simulink model "GFo_29bus"  (R2019a)
settings: Solver=ode1  StartTime=0.0  StopTime=4.5  FixedStep=Time_Step  RelTol=1e-3  EnableMultiTasking=on
PreLoadFcn:
  | Init_29bus;
InitFcn:
  | Init_29bus;
undefined symbols (not defined in the file): D1, D11, Delta, Time_Step, VSC01_Delta_P_Time_Step, VSC01_Delta_P_Value
libraries: powerlib x169, sps_avr x6, GFo_Lib x1
(part 1 of 5)
Description:
  | Copyright 2008-2017 The MathWorks, Inc.
settings Model: Creator=MathWorks  LastModifiedBy=fcolas
settings DataIOCC: SaveFormat=StructureWithTime  SignalLoggingSaveFormat=ModelDataLogs  SaveOutput=off  SignalLogging=off  DSMLogging=off  SaveTime=off  ReturnWorkspaceOutputs=off
settings OptimizationCC: ExpressionDepthLimit=2147483647  LifeSpan=inf
settings DebuggingCC: UnderspecifiedInitializationDetection=Classic  MergeDetectMultiDrivingBlocksExec=none  SolverPrmCheckMsg=warning  FcnCallInpInsideContextMsg=warning  UnconnectedInputMsg=none  UnconnectedOutputMsg=none  UnconnectedLineMsg=none  StateNameClashWarn=warning  SFUnexpectedBacktrackingDiag=warning  SFNoUnconditionalDefaultTransitionDiag=warning  SFExecutionAtInitializationDiag=none  ArithmeticOperatorsInVariantConditions=warning
settings HardwareCC: ProdBitPerPointer=32  ProdBitPerSizeT=32  ProdBitPerPtrDiffT=32  ProdLargestAtomicFloat=None  ProdIntDivRoundTo=Undefined  ProdEndianess=Unspecified  ProdWordSize=32  ProdHWDeviceType=32-bit Generic
settings ModelReferenceCC: PropagateSignalLabelsOutOfModel=off
settings SFSimCC: SimUseLocalCustomCode=off
settings RTWCC: RTWUseLocalCustomCode=off
settings CodeAppCC: StateflowObjectComments=on
settings GRTTargetCC: TargetLangStandard=C89/C90 (ANSI)  CombineOutputUpdateFcns=off  GRTInterface=on
settings ConfigComp: CovMetricSettings=dw  CovSaveCumulativeToWorkspaceVar=on  CovSaveSingleToWorkspaceVar=on  CovExternalEMLEnable=off  CovSFcnEnable=off
settings SimscapeCC: SimscapeNormalizeSystem=off

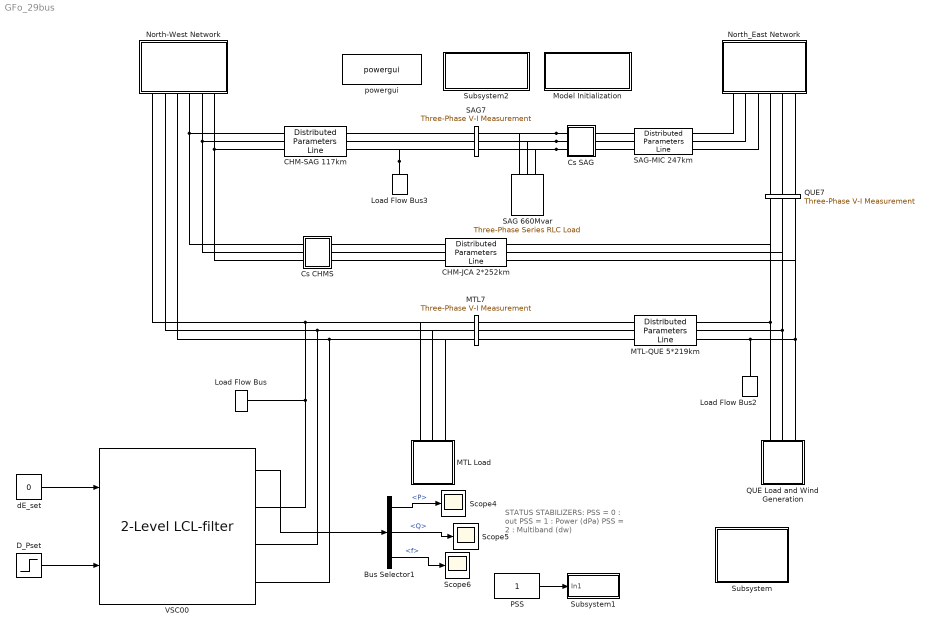
== system GFo_29bus ==
  note: STATUS STABILIZERS:
      | PSS = 0 :  out
      | PSS = 1 :  Power (dPa)
      | PSS = 2 :  Multiband (dw)
  Bus Selector1 : BusSelector  OutputSignals=P,Q,f
  CHM-JCA 2*252km : powerlib/Elements/Distributed Parameters Line  Phases=3  Length=252  Frequency=60  Resistance="[0.01273  0.3864]/2"  Inductance="[0.9337e-3  4.1264e-3]/2"  Capacitance=[12.74e-9 7.751e-9]*2  x1=[-0.00144 -3.19600605904016e-08 0 0;-0.0014 -3.19816909359179e-08 0 0;-0.00136 -3.19960489207136e-08 0 0;-0.00132 -3.2003131279907e-08 0 0;-0.00128 -3.20029364030306e-08 0 0;-0.00124 -3.19954643343978e-08 0 0;-0.0012 -3.19807167730924e-08 0 0;-0.00116 -3.19586970725827e-08 0 0;-0.00112 -3.19294102399589e-08 0 0;-0.00108 -3.18928629347939e-08 0 0;-0.00104 -3.184906346763e-08 0 0;-0.001 -3.17980217980881e-08 0 0;-0.00096 -3.17397495326038e-08 0 0;-0.00092 -3.16742599217877e-08 0 0;-0.00088 -3.16015678574126e-08 236947.551930455 -735006.025979769;-0.00084 -3.1521689869027e-08 248003.849356848 -731349.489711583;-0.0008 -3.14346441201967e-08 259003.752846592 -727526.650876326;-0.00076 -3.13404504043743e-08 269944.761116491 -723538.378754583;-0.00072 -3.12391301403984e-08 280824.386275617 -719385.58024504;-0.00068 -3.11307063676234e-08 291640.154391031 -715069.199658266;-0.00064 -3.10152037406802e-08 302389.606050334 -710590.218501984;-0.0006 -3.08926485238701e-08 313070.296920917 -705949.655257884;-0.00056 -3.07630685851926e-08 323679.798305784 -701148.565150029;-0.00052 -3.06264933900081e-08 334215.697695812 -696188.039904907;-0.00048 -3.04829539943384e-08 344675.599318338 -691069.207503179;-0.00044 -3.03324830378042e-08 355057.124681934 -685793.231923193;-0.0004 -3.01751147362034e-08 365357.913117259 -680361.312876297;-0.00036 -3.00108848737306e-08 375575.622313855 -674774.685534038;-0.00032 -2.98398307948405e-08 385707.928852762 -669034.620247298;-0.00028 -2.96619913957553e-08 395752.528734852 -663142.422257422;-0.00024 -2.94774071156208e-08 405707.137904732 -657099.431399422;-0.0002 -2.92861199273106e-08 415569.492770122 -650907.021797306;-0.00016 -2.90881733278817e-08 425337.350716574 -644566.601551616;-0.00012 -2.88836123286837e-08 435008.490617427 -638079.61241924;-8e-05 -2.86724834451239e-08 444580.713338866 -631447.529485563;-4e-05 -2.84548346860896e-08 454051.842239994 -624671.860829052]  x2=[-0.00144 -1.99708646271009e-08 0 0;-0.0014 -1.99485959351421e-08 0 0;-0.00136 -1.9921791104497e-08 0 0;-0.00132 -1.9890456230353e-08 0 0;-0.00128 -1.98545984379901e-08 0 0;-0.00124 -1.98142258811612e-08 0 0;-0.0012 -1.97693477402376e-08 0 0;-0.00116 -1.97199742201214e-08 0 0;-0.00112 -1.96661165479254e-08 0 0;-0.00108 -1.96077869704197e-08 0 0;-0.00104 -1.95449987512473e-08 0 0;-0.001 -1.94777661679078e-08 0 0;-0.00096 -1.94061045085108e-08 0 0;-0.00092 -1.93300300682997e-08 0 0;-0.00088 -1.92495601459461e-08 28167.8544791851 -750122.429836286;-0.00084 -1.91647130396165e-08 39475.8227942449 -749612.370451288;-0.0008 -1.90755080428111e-08 50774.8146476263 -748931.855677631;-0.00076 -1.8981965439977e-08 62062.2607460202 -748081.040258507;-0.00072 -1.88841065018953e-08 73335.5944215226 -747060.117662004;-0.00068 -1.87819534808447e-08 84592.2522152727 -745869.320037117;-0.00064 -1.86755296055411e-08 95829.6744603617 -744508.918160956;-0.0006 -1.85648590758562e-08 107045.305863878 -742979.221377177;-0.00056 -1.8449967057314e-08 118236.596087961 -741280.577525637;-0.00052 -1.83308796753687e-08 129401.000329722 -739413.372863299;-0.00048 -1.8207624009464e-08 140535.979899915 -737378.031976401;-0.00044 -1.80802280868754e-08 151639.002800209 -735175.017683909;-0.0004 -1.79487208763371e-08 162707.544298945 -732804.830932275;-0.00036 -1.78131322814546e-08 173739.087505238 -730268.010681527;-0.00032 -1.76734931339053e-08 184731.123941295 -727565.133782713;-0.00028 -1.75298351864271e-08 195681.15411282 -724696.814846731;-0.00024 -1.73821911055983e-08 206586.688077383 -721663.706104573;-0.0002 -1.72305944644097e-08 217445.246010605 -718466.497259008;-0.00016 -1.70750797346303e-08 228254.358770052 -715105.915327759;-0.00012 -1.69156822789684e-08 239011.568456696 -711582.724478174;-8e-05 -1.67524383430309e-08 249714.428973821 -707897.725853471;-4e-05 -1.65853850470811e-08 260360.506583243 -704051.757390559]  x3=[-0.00144 -7.69933611892035e-11 0 0;-0.0014 -7.64742706604721e-11 0 0;-0.00136 -7.59377905420784e-11 0 0;-0.00132 -7.53840428249751e-11 0 0;-0.00128 -7.48131534266176e-11 0 0;-0.00124 -7.42252521623322e-11 0 0;-0.0012 -7.36204727157963e-11 0 0;-0.00116 -7.29989526086407e-11 0 0;-0.00112 -7.23608331691782e-11 0 0;-0.00108 -7.17062595002662e-11 0 0;-0.00104 -7.10353804463122e-11 0 0;-0.001 -7.03483485594278e-11 0 0;-0.00096 -6.96453200647394e-11 0 0;-0.00092 -6.89264548248638e-11 0 0;-0.00088 -6.81919163035575e-11 329.831041715847 -923.135468477979;-0.00084 -6.74418715285459e-11 343.713540365703 -918.056958472584;-0.0008 -6.66764910535426e-11 357.517881520539 -912.769690231818;-0.00076 -6.58959489194672e-11 371.24092619222 -907.274866034884;-0.00072 -6.51004226148701e-11 384.87955387873 -901.573735357418;-0.00068 -6.42900930355724e-11 398.430663273748 -895.667594587374;-0.00064 -6.34651444435326e-11 411.891172971858 -889.557786730228;-0.0006 -6.26257644249465e-11 425.258022169232 -883.2457011036;-0.00056 -6.17721438475917e-11 438.528171359633 -876.732773021327;-0.00052 -6.09044768174262e-11 451.698603025574 -870.020483467091;-0.00048 -6.00229606344503e-11 464.766322324469 -863.110358757651;-0.00044 -5.91277957478421e-11 477.728357769642 -856.003970195776;-0.0004 -5.82191857103772e-11 490.581761906011 -848.702933712943;-0.00036 -5.72973371321427e-11 503.32361198032 -841.208909501886;-0.00032 -5.63624596335555e-11 515.951010605743 -833.523601639085;-0.00028 -5.54147657976968e-11 528.461086420726 -825.648757697273;-0.00024 -5.44544711219723e-11 540.850994741912 -817.586168348051;-0.0002 -5.348179396911e-11 553.117918210993 -809.337666954711;-0.00016 -5.24969555175064e-11 565.259067435359 -800.905129155335;-0.00012 -5.15001797109327e-11 577.271681622377 -792.290472436302;-8e-05 -5.04916932076113e-11 589.153029207173 -783.495655696258;-4e-05 -4.94717253286763e-11 600.900408473766 -774.522678800688]  x4=[-0.00144 -4.78587088598672e-11 0 0;-0.0014 -4.8966645663073e-11 0 0;-0.00136 -5.00634478733254e-11 0 0;-0.00132 -5.11488660872601e-11 0 0;-0.00128 -5.22226534901357e-11 0 0;-0.00124 -5.32845659119566e-11 0 0;-0.0012 -5.43343618829956e-11 0 0;-0.00116 -5.5371802688702e-11 0 0;-0.00112 -5.63966524239831e-11 0 0;-0.00108 -5.7408678046847e-11 0 0;-0.00104 -5.84076494313944e-11 0 0;-0.001 -5.93933394201472e-11 0 0;-0.00096 -6.03655238757023e-11 0 0;-0.00092 -6.13239817316981e-11 0 0;-0.00088 -6.22684950430836e-11 -191.737879033599 -10272.54825288;-0.00084 -6.31988490356769e-11 -36.8152546194894 -10274.2711335707;-0.0008 -6.41148321550032e-11 118.115741266039 -10273.6577336072;-0.00076 -6.50162361144002e-11 273.019878650591 -10270.7081924713;-0.00072 -6.59028559423809e-11 427.861933669161 -10265.4231808633;-0.00068 -6.67744900292424e-11 582.606696573739 -10257.8039005491;-0.00064 -6.76309401729099e-11 737.218979739702 -10247.8520840876;-0.0006 -6.84720116240064e-11 891.663625667178 -10235.5699944358;-0.00056 -6.92975131301371e-11 1045.90551497556 -10220.960424435;-0.00052 -7.01072569793784e-11 1199.90957438934 -10204.0266961756;-0.00048 -7.09010590429617e-11 1353.64078471348 -10184.7726602412;-0.00044 -7.16787388171434e-11 1507.06418879648 -10163.2026948337;-0.0004 -7.24401194642492e-11 1660.14489947931 -10139.321704777;-0.00036 -7.31850278528858e-11 1812.84810752848 -10113.1351204025;-0.00032 -7.39132945973095e-11 1965.13908955134 -10084.6488963136;-0.00028 -7.46247540959428e-11 2116.98321589187 -10053.8695100319;-0.00024 -7.53192445690312e-11 2268.3459585052 -10020.8039605246;-0.0002 -7.59966080954301e-11 2419.19289880894 -9985.45976661232;-0.00016 -7.66566906485149e-11 2569.48973550972 -9947.84496526009;-0.00012 -7.72993421312054e-11 2719.20229240298 -9907.96810974931;-8e-05 -7.79244164100964e-11 2868.29652614436 -9865.83826773306;-4e-05 -7.85317713486873e-11 3016.73853399082 -9821.46501917409]  x5=0.00142516474882927  V1=ones(3,3)  V2=ones(3,3)  I1=ones(3,3)  I2=ones(3,3)  nHarmo=1  Measurements=None  Decoupling=off  VsMag0=0  VrMag0=0  VsAngle0=0  VrAngle0=0  IsMag0=0  IrMag0=0  IsAngle0=0  IrAngle0=0
      settings: AttributesFormatString=\n
  CHM-SAG 117km : powerlib/Elements/Distributed Parameters Line  Phases=3  Length=117  Frequency=60  Resistance="[0.01273  0.3864]"  Inductance="[0.9337e-3  4.1264e-3]"  Capacitance=[12.74e-9 7.751e-9]  x1=[-0.00068 -3.03380786364724e-08 0 0;-0.00064 -3.02440322105761e-08 0 0;-0.0006 -3.01431085525686e-08 0 0;-0.00056 -3.00353306116193e-08 0 0;-0.00052 -2.99207228955026e-08 0 0;-0.00048 -2.97993114650248e-08 0 0;-0.00044 -2.96711239280981e-08 285915.250875642 -721016.735543736;-0.0004 -2.95361894334631e-08 296755.036613392 -716623.402960289;-0.00036 -2.93945386640601e-08 307527.342814922 -712067.116394906;-0.00032 -2.92462038300527e-08 318229.719950699 -707348.911907859;-0.00028 -2.90912186615028e-08 328859.734392455 -702469.862378162;-0.00024 -2.89296184007012e-08 339414.968966577 -697431.077259603;-0.0002 -2.87614397941538e-08 349893.023503745 -692233.702328464;-0.00016 -2.85867210842252e-08 360291.515384717 -686878.919422984;-0.00012 -2.84055020004435e-08 370608.080082112 -681367.94617462;-8e-05 -2.82178237504655e-08 380840.371698085 -675702.035731162;-4e-05 -2.80237290107068e-08 390986.063497761 -669882.476471785]  x2=[-0.00068 -2.03559263742575e-08 0 0;-0.00064 -2.02730116097309e-08 0 0;-0.0006 -2.01854869371913e-08 0 0;-0.00056 -2.00933722589944e-08 0 0;-0.00052 -1.99966885212236e-08 0 0;-0.00048 -1.98954577089273e-08 0 0;-0.00044 -1.9789702841119e-08 332776.301409875 -689011.544371815;-0.0004 -1.96794479655438e-08 343128.151600731 -683915.224593623;-0.00036 -1.95647181532096e-08 353401.977408923 -678663.388391192;-0.00032 -1.94455394926862e-08 363595.442655062 -673257.229986786;-0.00028 -1.93219390841734e-08 373706.229433054 -667697.978694203;-0.00024 -1.91939450333382e-08 383732.038637179 -661986.898639247;-0.0002 -1.9061586444924e-08 393670.590484882 -656125.288472272;-0.00016 -1.89248934161323e-08 403519.625035179 -650114.481072883;-0.00012 -1.8783897029779e-08 413276.902702548 -643955.843246846;-8e-05 -1.86386293472267e-08 422940.204766191 -637650.775415293;-4e-05 -1.84891234010935e-08 432507.333874551 -631200.711296277]  x3=[-0.00068 -2.53056281828965e-11 0 0;-0.00064 -2.45024672055226e-11 0 0;-0.0006 -2.36937345784065e-11 0 0;-0.00056 -2.28796142003733e-11 0 0;-0.00052 -2.20602911953763e-11 0 0;-0.00048 -2.12359518704014e-11 0 0;-0.00044 -2.04067836731021e-11 1667.28750300292 -3842.30394709011;-0.0004 -1.95729751491762e-11 1725.03630670092 -3816.72583715085;-0.00036 -1.87347158994916e-11 1782.39285201884 -3790.27983667027;-0.00032 -1.78921965369727e-11 1839.34409657292 -3762.97195924081;-0.00028 -1.7045608643257e-11 1895.87709014127 -3734.80841443831;-0.00024 -1.61951447251309e-11 1951.97897760867 -3705.79560640998;-0.0002 -1.53409981707553e-11 2007.6370018897 -3675.94013241817;-0.00016 -1.44833632056908e-11 2062.83850682964 -3645.24878134021;-0.00012 -1.36224348487326e-11 2117.57094008228 -3613.72853212466;-8e-05 -1.27584088675646e-11 2171.8218559643 -3581.38655220437;-4e-05 -1.1891481734244e-11 2225.57891828527 -3548.23019586668]  x4=[-0.00068 -4.55030209021528e-11 0 0;-0.00064 -4.62034510762418e-11 0 0;-0.0006 -4.68933749839977e-11 0 0;-0.00056 -4.75726357426735e-11 0 0;-0.00052 -4.82410788942303e-11 0 0;-0.00048 -4.88985524404599e-11 0 0;-0.00044 -4.95449068775477e-11 212.800113436249 -1518.35731015853;-0.0004 -5.01799952300687e-11 235.671559779652 -1514.9757824875;-0.00036 -5.08036730844081e-11 258.489416442706 -1511.24976238813;-0.00032 -5.14157986216004e-11 281.248494841579 -1507.18009712526;-0.00028 -5.20162326495771e-11 303.943619758109 -1502.76771210566;-0.00024 -5.26048386348182e-11 326.569630516604 -1498.01361066765;-0.0002 -5.31814827333985e-11 349.121382157336 -1492.9188738529;-0.00016 -5.37460338214228e-11 371.59374660646 -1487.48466016061;-0.00012 -5.42983635248422e-11 393.981613842093 -1481.71220528413;-8e-05 -5.48383462486452e-11 416.279893056292 -1475.6028218299;-4e-05 -5.5365859205417e-11 438.483513812655 -1469.15789901905]  x5=0.000661683633385019  V1=ones(3,3)  V2=ones(3,3)  I1=ones(3,3)  I2=ones(3,3)  nHarmo=1  Measurements=None  Decoupling=off  VsMag0=0  VrMag0=0  VsAngle0=0  VrAngle0=0  IsMag0=0  IrMag0=0  IsAngle0=0  IrAngle0=0
      settings: AttributesFormatString=\n
  Cs CHMS : Subsystem  mask{Xc=33/2}
      mask prompts: Xc "Condensator Reactance at  60Hz  (ohm):"
      mask help: Series Compensation
      mask init:
      | Cs=1/Xc/(2*pi*60);
      mask Display: disp('Cs')
  Cs SAG : Subsystem  mask{Xc=22}
      mask prompts: Xc "Condensator Reactance at  60Hz  (ohm):"
      mask help: Series Compensation
      mask init:
      | Cs=1/Xc/(2*pi*60);
      mask Display: disp('Cs')
  D_Pset : Step  Time=VSC01_Delta_P_Time_Step  After=VSC01_Delta_P_Value  SampleTime=0
  Load Flow Bus : powerlib/Measurements/Load Flow Bus  LConnTagsString=a  Phases=single  Connectors=on one side  ID=BUS_1  Vbase=VSC01_Un2  Vref=1  Vangle=0  VLF=1  VLFb=1  VLFc=1  angleLF=-17.01  angleLFb=0  angleLFc=0
  Load Flow Bus2 : powerlib/Measurements/Load Flow Bus  LConnTagsString=a  Phases=single  Connectors=on one side  ID=QUE7  Vbase=735e3  Vref=1  Vangle=0  VLF=1.021  VLFb=1  VLFc=1  angleLF=-8.842  angleLFb=0  angleLFc=0
      settings: AttributesFormatString=%<ID>\n%<Vbase>V\n%<VLF>pu\n%<angleLF>deg.
  Load Flow Bus3 : powerlib/Measurements/Load Flow Bus  LConnTagsString=a  Phases=single  Connectors=on one side  ID=SAG7  Vbase=735e3  Vref=1  Vangle=0  VLF=1.041  VLFb=1  VLFc=1  angleLF=5.283  angleLFb=0  angleLFc=0
      settings: AttributesFormatString=%<ID>\n%<Vbase>V\n%<VLF>pu\n%<angleLF>deg.
  MTL Load : Subsystem
  MTL-QUE 5*219km : powerlib/Elements/Distributed Parameters Line  Phases=3  Length=219  Frequency=60  Resistance="[0.01273  0.3864]/5"  Inductance="[0.9337e-3  4.1264e-3]/5"  Capacitance=[12.74e-9 7.751e-9]*5  x1=[-0.00124 -1.25867854068197e-07 -175262.845803513 -713799.758659387;-0.0012 -1.25881992959478e-07 -164479.469159206 -716361.379291285;-0.00116 -1.25867507371121e-07 -153658.691302023 -718760.10552317;-0.00112 -1.25824400597023e-07 -142802.972783534 -720995.391905382;-0.00108 -1.25752682439292e-07 -131914.782100514 -723066.730153074;-0.00104 -1.2565236920602e-07 -120996.59513363 -724973.649261791;-0.001 -1.2552348370757e-07 -110050.894584442 -726715.715614573;-0.00096 -1.25366055251394e-07 -99080.1694108641 -728292.533080553;-0.00092 -1.25180119635364e-07 -88086.9142611932 -729703.743105038;-0.00088 -1.24965719139636e-07 -77073.6289068485 -730949.024791039;-0.00084 -1.24722902517035e-07 -66042.8176739451 -732028.094972237;-0.0008 -1.24451724981965e-07 -54996.9888738316 -732940.70827738;-0.00076 -1.24152248197861e-07 -43938.6542327221 -733686.657186073;-0.00072 -1.2382454026316e-07 -32870.3283205508 -734265.772075965;-0.00068 -1.2346867569582e-07 -21794.5279791811 -734677.921261326;-0.00064 -1.23084735416376e-07 -10713.7717500969 -734923.011022985;-0.0006 -1.22672806729535e-07 369.420698291617 -735000.985629643;-0.00056 -1.2223298330433e-07 11452.5291435991 -734911.827350547;-0.00052 -1.21765365152813e-07 22533.0333825417 -734655.556459522;-0.00048 -1.21270058607321e-07 33608.4138040097 -734232.231230357;-0.00044 -1.20747176296289e-07 44676.1519620054 -733641.94792356;-0.0004 -1.20196837118647e-07 55733.7311483156 -732884.840764464;-0.00036 -1.19619166216778e-07 66778.6369647899 -731961.081912707;-0.00032 -1.19014294948063e-07 77808.3578950928 -730870.881423087;-0.00028 -1.18382360855012e-07 88820.3858758011 -729614.487197794;-0.00024 -1.17723507633989e-07 99812.2168667156 -728192.184930039;-0.0002 -1.17037885102534e-07 110781.351420259 -726604.298039093;-0.00016 -1.16325649165298e-07 121725.295249826 -724851.187596741;-0.00012 -1.15586961778592e-07 132641.559796968 -722933.25224518;-8e-05 -1.14821990913557e-07 143527.662797265 -720850.92810637;-4e-05 -1.14030910517971e-07 154381.128844771 -718604.688682862]  x2=[-0.00124 -1.98142258811612e-08 -73583.3206392189 -747036.13816367;-0.0012 -1.97693477402376e-08 -62310.3261187054 -748060.740678712;-0.00116 -1.97199742201214e-08 -51023.1627673739 -748915.240632326;-0.00112 -1.96661165479254e-08 -39724.3971888341 -749599.443718591;-0.00108 -1.96077869704197e-08 -28416.5986249423 -750113.194355623;-0.00104 -1.95449987512473e-08 -17102.3383715773 -750456.37572096;-0.001 -1.94777661679078e-08 -5784.18919395105 -750628.909778118;-0.00096 -1.94061045085108e-08 5535.27525841725 -750630.757294341;-0.00092 -1.93300300682997e-08 16853.481036926 -750461.917849519;-0.00088 -1.92495601459461e-08 28167.8544791852 -750122.429836286;-0.00084 -1.91647130396165e-08 39475.8227942449 -749612.370451288;-0.0008 -1.90755080428111e-08 50774.8146476264 -748931.855677631;-0.00076 -1.8981965439977e-08 62062.2607460202 -748081.040258507;-0.00072 -1.88841065018953e-08 73335.5944215226 -747060.117662004;-0.00068 -1.87819534808447e-08 84592.2522152728 -745869.320037117;-0.00064 -1.86755296055411e-08 95829.6744603617 -744508.918160956;-0.0006 -1.85648590758562e-08 107045.305863878 -742979.221377177;-0.00056 -1.8449967057314e-08 118236.596087961 -741280.577525637;-0.00052 -1.83308796753687e-08 129401.000329722 -739413.372863299;-0.00048 -1.8207624009464e-08 140535.979899915 -737378.031976401;-0.00044 -1.80802280868754e-08 151639.002800209 -735175.017683909;-0.0004 -1.79487208763371e-08 162707.544298945 -732804.830932275;-0.00036 -1.78131322814546e-08 173739.087505238 -730268.010681527;-0.00032 -1.76734931339053e-08 184731.123941295 -727565.133782713;-0.00028 -1.75298351864271e-08 195681.15411282 -724696.814846731;-0.00024 -1.73821911055983e-08 206586.688077383 -721663.706104573;-0.0002 -1.72305944644097e-08 217445.246010605 -718466.497259008;-0.00016 -1.70750797346303e-08 228254.358770052 -715105.915327759;-0.00012 -1.69156822789684e-08 239011.568456696 -711582.724478174;-8e-05 -1.67524383430309e-08 249714.428973821 -707897.725853471;-4e-05 -1.65853850470811e-08 260360.506583243 -704051.757390559]  x3=[-0.00124 -5.10144217917009e-10 -7027.03988727101 -19339.1228874643;-0.0012 -4.91343394355244e-10 -6734.62515238683 -19442.8845645399;-0.00116 -4.72430843542768e-10 -6440.67902181993 -19542.2250973339;-0.00112 -4.53410866030541e-10 -6145.26833638552 -19637.1218966656;-0.00108 -4.34287786797427e-10 -5848.46026992595 -19727.5533838215;-0.00104 -4.15065954266734e-10 -5550.32231403597 -19813.4989954609;-0.001 -3.95749739317417e-10 -5250.92226271573 -19894.9391882932;-0.00096 -3.76343534290179e-10 -4950.32819695497 -19971.8554435207;-0.00092 -3.56851751988693e-10 -4648.60846925203 -20044.2302710503;-0.00088 -3.37278824676162e-10 -4345.83168807107 -20112.0472134703;-0.00084 -3.17629203067469e-10 -4042.06670224111 -20175.2908497929;-0.0008 -2.97907355317116e-10 -3737.38258530035 -20233.9467989606;-0.00076 -2.78117766003207e-10 -3431.84861978952 -20288.0017231163;-0.00072 -2.58264935107695e-10 -3125.53428149754 -20337.4433306364;-0.00068 -2.38353376993122e-10 -2818.50922366341 -20382.2603789258;-0.00064 -2.18387619376091e-10 -2510.84326113761 -20422.4426769741;-0.0006 -1.9837220229771e-10 -2202.60635450682 -20457.9810876734;-0.00056 -1.78311677091215e-10 -1893.86859418547 -20488.8675298954;-0.00052 -1.58210605347044e-10 -1584.70018447784 -20515.0949803296;-0.00048 -1.38073557875567e-10 -1275.17142761413 -20536.6574750799;-0.00044 -1.17905113667725e-10 -965.352707764394 -20553.550111021;-0.0004 -9.77098588538048e-11 -655.314475033757 -20565.7690469131;-0.00036 -7.74923856605955e-11 -345.127229442688 -20573.3115042756;-0.00032 -5.72572913671529e-11 -34.8615048958939 -20576.1757680186;-0.00028 -3.70091772594193e-11 275.41214685648 -20574.3611868334;-0.00024 -1.67526475839304e-11 585.623172261712 -20567.8681733401;-0.0002 3.50769149915035e-12 895.701032007771 -20556.6982039939;-0.00016 2.37672329634333e-11 1205.57521706335 -20540.8538187495;-0.00012 4.40213699639002e-11 1515.175264711 -20520.3386204835;-8e-05 6.42654968844614e-11 1824.43077456978 -20495.1572741751;-4e-05 8.44950103852332e-11 2133.27142460364 -20465.3155058452]  x4=[-0.00124 -4.08867860944578e-10 -1381.07232417721 -6777.19407549483;-0.0012 -4.30955175950684e-10 -1278.7208894892 -6797.24853422087;-0.00116 -4.52944495466178e-10 -1176.07868469815 -6815.7573572472;-0.00112 -4.74830819309429e-10 -1073.16904975626 -6832.71633582708;-0.00108 -4.96609170719137e-10 -970.015385427081 -6848.12161363503;-0.00104 -5.18274597485997e-10 -866.641147964308 -6861.96968764373;-0.001 -5.398221730788e-10 -763.069843778083 -6874.25740892056;-0.00096 -5.61246997764672e-10 -659.325024089817 -6884.98198334367;-0.00092 -5.82544199723241e-10 -555.43027957685 -6894.14097223733;-0.00088 -6.03708936154439e-10 -451.409235008133 -6901.73229292644;-0.00084 -6.24736394379721e-10 -347.285543872164 -6907.75421921014;-0.0008 -6.45621792936417e-10 -243.08288299838 -6912.20538175433;-0.00076 -6.66360382665005e-10 -138.824947173261 -6915.08476840304;-0.00072 -6.86947447789023e-10 -34.5354437523297 -6916.39172440855;-0.00068 -7.07378306987395e-10 69.76191273069 -6916.12595258036;-0.00064 -7.27648314458929e-10 174.043405956356 -6914.28751335268;-0.0006 -7.47752860978728e-10 278.285323212394 -6910.87682477074;-0.00056 -7.67687374946285e-10 382.463960785763 -6905.89466239571;-0.00052 -7.87447323425034e-10 486.555629352679 -6899.34215912835;-0.00048 -8.07028213173093e-10 590.536659365357 -6891.2208049514;-0.00044 -8.2642559166499e-10 694.383406434267 -6881.53244659076;-0.0004 -8.45635048104134e-10 798.072256704661 -6870.27928709557;-0.00036 -8.64652214425785e-10 901.579632226162 -6857.46388533727;-0.00032 -8.8347276629032e-10 1004.88199631419 -6843.08915542768;-0.00028 -9.02092424066543e-10 1107.95585890198 -6827.15836605644;-0.00024 -9.20506953804849e-10 1210.77778188207 -6809.67513974767;-0.0002 -9.38712168199972e-10 1313.32438443586 -6790.64345203625;-0.00016 -9.56703927543156e-10 1415.57234835025 -6770.06763056386;-0.00012 -9.7447814066348e-10 1517.49842332001 -6747.95235409485;-8e-05 -9.92030765858159e-10 1619.07943223465 -6724.30265145239;-4e-05 -1.00935781181159e-09 1720.29227644875 -6699.1239003749]  x5=0.00123853603172068  V1=ones(3,3)  V2=ones(3,3)  I1=ones(3,3)  I2=ones(3,3)  nHarmo=1  Measurements=None  Decoupling=off  VsMag0=0  VrMag0=0  VsAngle0=0  VrAngle0=0  IsMag0=0  IrMag0=0  IsAngle0=0  IrAngle0=0
      settings: AttributesFormatString=\n
  MTL7 : powerlib/Measurements/Three-Phase V-I Measurement  VoltageMeasurement=phase-to-ground  SetLabelV=on  LabelV=Vabc_MTL7  Vpu=on  VpuLL=off  CurrentMeasurement=no  SetLabelI=off  LabelI=A1  Ipu=off  Pbase=100e6  Vbase=735e3  OutputType=Magnitude  PhasorSimulation=off  PSBequivalent=0
  Model Initialization : Subsystem  mask(Model Functions){InitFcnX=Init_29bus;, prel=on, posl=off, inif=on, strf=off}
      mask prompts: InitFcnX "Initialisation"; prel "Preload Function"; posl "PostLoad Function"; inif "InitFcn"; strf "StartFcn"
      mask init:
      | currentBlock = gcb;
      | root = bdroot(currentBlock);
      | 
      | if ~strcmp(get_param(root,'BlockDiagramType'),'library')
      |     if prel==1
      |         set_param(root, 'PreLoadFcn', InitFcnX);
      |     else
      |         set_param(root, 'PreLoadFcn', '');
      |     end
      |     if inif==1
      |         set_param(root, 'InitFcn', InitFcnX);
      |     else
      |         set_param(root, 'InitFcn', '');
      |     end
      |     if strf==1
      |         set_param(root, 'StartFcn', InitFcnX);
      |     else
      |         set_param(root, 'StartFcn', '');
      |     end
      |     if posl==1
      |         set_param(root, 'PostLoadFcn', InitFcnX);
      |     else
      |         set_param(root, 'PostLoadFcn', '');
      |     end
      | end
      | 
      | pos = get_param(currentBlock, 'Position');
      | width = pos(3) - pos(1); height = pos(4) - pos(2);
      | txt = [ upper(root) '\n' '- InitFcn. . . . . '  get_param(root, 'InitFcn') ];
      settings: CopyFcn=set_param(gcb,'LinkStatus','none')
      mask Display:
      | %text(5, height*0.5, txt, 'horizontalAlignment', 'left', 'verticalAlignment', 'middle') ;
      | color('blue'),disp('Initialization Function\nParameters')
  North-West Network : Subsystem
  North_East Network : Subsystem
  PSS : Constant
  QUE Load and Wind Generation : Subsystem
  QUE7 : powerlib/Measurements/Three-Phase V-I Measurement  VoltageMeasurement=no  SetLabelV=on  LabelV=Vabc_QUE7  Vpu=on  VpuLL=off  CurrentMeasurement=no  SetLabelI=off  LabelI=A1  Ipu=off  Pbase=100e6  Vbase=735e3  OutputType=Magnitude  PhasorSimulation=off  PSBequivalent=0
  SAG 660Mvar : powerlib/Elements/Three-Phase Series RLC Load  LConnTagsString=A|B|C  Configuration=Y (grounded)  NominalVoltage=735e3  Vabc=[1e3 1e3 1e3]  Vabcp=[1e3 1e3 1e3]  NominalFrequency=60  UnbalancedPower=off  ActivePower=2200000  InductivePower=660e6  CapacitivePower=0  Pabc=[10e3 9e3 11e3]  QLabc=[100 90 110]  QCabc=[100 90 110]  Pabcp=[10e3 9e3 11e3]  QLabcp=[100 90 110]  QCabcp=[100 90 110]  Measurements=None  LoadType=constant Z
  SAG-MIC 247km : powerlib/Elements/Distributed Parameters Line  Phases=3  Length=247  Frequency=60  Resistance="[0.01273  0.3864]/1"  Inductance="[0.9337e-3  4.1264e-3]/1"  Capacitance=[12.74e-9 7.751e-9]*1  x1=[-0.0014 -2.0715212238375e-08 36522.5847829561 -754650.708753614;-0.00136 -2.07364597068543e-08 47897.8850362566 -754014.151844709;-0.00132 -2.07529918832199e-08 59262.2937235537 -753206.138620016;-0.00128 -2.07648050081973e-08 70613.2266763144 -752226.852814774;-0.00124 -2.0771896395584e-08 81948.1027902712 -751076.51711013;-0.0012 -2.07742644328595e-08 93264.3446123441 -749755.393082503;-0.00116 -2.07719085815526e-08 104559.378926729 -748263.781144104;-0.00112 -2.07648293773636e-08 115830.637340029 -746602.020474625;-0.00108 -2.07530284300425e-08 127075.556865277 -744770.488944111;-0.00104 -2.07365084230228e-08 138291.580504748 -742769.603027039;-0.001 -2.07152731128118e-08 149476.157831388 -740599.817707611;-0.00096 -2.06893273281358e-08 160626.745568764 -738261.626376297;-0.00092 -2.06586769688425e-08 171740.808169384 -735755.560717642;-0.00088 -2.06233290045594e-08 182815.818391256 -733082.190589366;-0.00084 -2.05832914731087e-08 193849.257872562 -730242.123892781;-0.0008 -2.05385734786797e-08 204838.617704313 -727236.006434563;-0.00076 -2.04891851897588e-08 215781.399000851 -724064.521779898;-0.00072 -2.0435137836817e-08 226675.113468075 -720728.391097046;-0.00068 -2.03764437097562e-08 237517.28396926 -717228.372993356;-0.00064 -2.03131161551147e-08 248305.445088332 -713565.263342761;-0.0006 -2.02451695730325e-08 259037.143690486 -709739.895104807;-0.00056 -2.01726194139762e-08 269709.939480006 -705753.138135243;-0.00052 -2.00954821752264e-08 280321.405555168 -701605.898988222;-0.00048 -2.00137753971261e-08 290869.128960095 -697299.120710163;-0.00044 -1.99275176590919e-08 301350.711233445 -692833.782625306;-0.0004 -1.98367285753896e-08 311763.768953799 -688210.900113024;-0.00036 -1.9741428790674e-08 322105.934281629 -683431.524376934;-0.00032 -1.96416399752941e-08 332374.855497726 -678496.742205864;-0.00028 -1.95373848203662e-08 342568.197537962 -673407.675726722;-0.00024 -1.94286870326134e-08 352683.64252426 -668165.482149341;-0.0002 -1.93155713289752e-08 362718.890291662 -662771.353503333;-0.00016 -1.91980634309872e-08 372671.658911367 -657226.516367035;-0.00012 -1.9076190058932e-08 382539.685209618 -651532.231588595;-8e-05 -1.89499789257635e-08 392320.725282335 -645689.793999266;-4e-05 -1.88194587308049e-08 402012.555005352 -639700.532118974]  x2=[-0.0014 -8.27139318429975e-09 154421.725077414 -749560.143874635;-0.00136 -8.30049042152564e-09 165706.858590059 -747146.344688553;-0.00132 -8.32770019881005e-09 176954.311792055 -744562.650866804;-0.00128 -8.35301632888428e-09 188161.527109539 -741809.649919084;-0.00124 -8.37643305507867e-09 199325.956118394 -738887.967854065;-0.0012 -8.39794505263161e-09 210445.060123741 -735798.269037055;-0.00116 -8.41754742990038e-09 221516.310737217 -732541.25603892;-0.00112 -8.43523572947343e-09 232537.190451907 -729117.669476329;-0.00108 -8.45100592918398e-09 243505.193214803 -725528.287843341;-0.00104 -8.46485444302459e-09 254417.824996662 -721773.927334388;-0.001 -8.47677812196266e-09 265272.604359122 -717855.441658672;-0.00096 -8.48677425465641e-09 276067.063018965 -713773.721846044;-0.00092 -8.49484056807148e-09 286798.746409378 -709529.696044391;-0.00088 -8.50097522799776e-09 297465.214238104 -705124.329308581;-0.00084 -8.50517683946648e-09 308064.041042344 -700558.62338102;-0.0008 -8.50744444706742e-09 318592.816740282 -695833.616463862;-0.00076 -8.50777753516618e-09 329049.14717912 -690950.382982933;-0.00072 -8.50617602802139e-09 339430.654679489 -685910.033343417;-0.00068 -8.50264028980196e-09 349734.978576109 -680713.713677354;-0.00064 -8.49717112450428e-09 359959.775754587 -675362.605583027;-0.0006 -8.48976977576937e-09 370102.721184219 -669857.925856268;-0.00056 -8.48043792660011e-09 380161.508446684 -664200.926213779;-0.00052 -8.46917769897852e-09 390133.850260501 -658392.893008494;-0.00048 -8.45599165338326e-09 400017.47900114 -652435.146937077;-0.00044 -8.44088278820739e-09 409810.147216658 -646329.042739607;-0.0004 -8.42385453907655e-09 419509.628138751 -640075.968891523;-0.00036 -8.40491077806776e-09 429113.716189102 -633677.347287893;-0.00032 -8.38405581282889e-09 438620.227480911 -627134.632920091;-0.00028 -8.3612943855992e-09 448027.000315491 -620449.313544941;-0.00024 -8.33663167213097e-09 457331.895673819 -613622.909346418;-0.0002 -8.31007328051254e-09 466532.797702933 -606656.972589968;-0.00016 -8.28162524989314e-09 475627.614197057 -599553.087269538;-0.00012 -8.25129404910961e-09 484614.277073351 -592312.868747389;-8e-05 -8.21908657521544e-09 493490.742842173 -584937.963386775;-4e-05 -8.18501015191245e-09 502254.993071756 -577430.048177577]  x3=[-0.0014 -1.78924563946058e-11 -207.547752866833 -4152.7477084931;-0.00136 -1.75997703945032e-11 -144.904646865292 -4155.40507498295;-0.00132 -1.73030823583868e-11 -82.2285907966585 -4157.11753819343;-0.00128 -1.70024597505576e-11 -19.5338366555868 -4157.88470872519;-0.00124 -1.66979709300041e-11 43.1653593114872 -4157.70641213025;-0.0012 -1.63896851348582e-11 105.854739848097 -4156.58268895172;-0.00116 -1.60776724666513e-11 168.520049929717 -4154.51379471457;-0.00112 -1.57620038743735e-11 231.147040005238 -4151.50019986751;-0.00108 -1.54427511383403e-11 293.721469237189 -4147.542589676;-0.00104 -1.51199868538709e-11 356.229108739981 -4142.64186406649;-0.001 -1.47937844147802e-11 418.655744815435 -4136.79913742171;-0.00096 -1.44642179966896e-11 480.987182184852 -4130.01573832732;-0.00092 -1.41313625401608e-11 543.209247216896 -4122.29320926977;-0.00088 -1.3795293733654e-11 605.307791150561 -4113.63330628557;-0.00084 -1.34560879963177e-11 667.268693312469 -4104.03799856199;-0.0008 -1.31138224606114e-11 729.077864327799 -4093.50946798926;-0.00076 -1.27685749547663e-11 790.72124932408 -4082.05010866442;-0.00072 -1.2420423985088e-11 852.184831127155 -4069.66252634697;-0.00068 -1.20694487181047e-11 913.45463344856 -4056.34953786631;-0.00064 -1.17157289625654e-11 974.516724063616 -4042.11417048121;-0.0006 -1.13593451512922e-11 1035.3572179795 -4026.95966119144;-0.00056 -1.10003783228903e-11 1095.96228059255 -4010.88945600175;-0.00052 -1.06389101033211e-11 1156.31813083417 -3993.90720913819;-0.00048 -1.02750226873404e-11 1216.4110443045 -3976.01678221727;-0.00044 -9.90879881980864e-12 1276.22735639323 -3957.22224336777;-0.0004 -9.54032177687509e-12 1335.75346538684 -3937.52786630577;-0.00036 -9.16967534704172e-12 1394.97583556147 -3916.93812936277;-0.00032 -8.79694381211034e-12 1453.88100026085 -3895.45771446738;-0.00028 -8.4222119280177e-12 1512.45556495851 -3873.09150608072;-0.00024 -8.04556490556269e-12 1570.68621030356 -3849.84459008569;-0.0002 -7.66708839103015e-12 1628.55969514941 -3825.72225263053;-0.00016 -7.28686844671565e-12 1686.06285956467 -3800.72997892674;-0.00012 -6.90499153135564e-12 1743.18262782567 -3774.87345200184;-8e-05 -6.52154448046751e-12 1799.90601138966 -3748.15855140708;-4e-05 -6.13661448660393e-12 1856.22011184838 -3720.59135188047]  x4=[-0.0014 -1.89201204911383e-11 11.9349515108093 -1468.59968146629;-0.00136 -1.94615873981848e-11 34.0788908853198 -1468.2525709345;-0.00132 -1.99986289080864e-11 56.215081013927 -1467.57159242976;-0.00128 -2.05311229022353e-11 78.3384883178897 -1466.55690080069;-0.00124 -2.1058948296089e-11 100.444082125171 -1465.20872677942;-0.0012 -2.15819850667048e-11 122.526835814371 -1463.52737692911;-0.00116 -2.21001142800316e-11 144.581727957732 -1461.51323357421;-0.00112 -2.26132181179543e-11 166.603743462976 -1459.16675471355;-0.00108 -2.31211799050851e-11 188.587874713685 -1456.48847391618;-0.00104 -2.36238841352941e-11 210.529122707997 -1453.47900020007;-0.001 -2.41212164979744e-11 232.422498195332 -1450.13901789358;-0.00096 -2.46130639040356e-11 254.263022810903 -1446.46928647989;-0.00092 -2.5099314511619e-11 276.045730207757 -1442.47064042427;-0.00088 -2.55798577515297e-11 297.76566718608 -1438.14398898436;-0.00084 -2.60545843523791e-11 319.417894819506 -1433.49031600337;-0.0008 -2.65233863654318e-11 340.997489578193 -1428.51067968642;-0.00076 -2.69861571891531e-11 362.499544448386 -1423.20621235987;-0.00072 -2.74427915934482e-11 383.919170048236 -1417.57812021383;-0.00068 -2.78931857435915e-11 405.251495739594 -1411.62768302792;-0.00064 -2.83372372238373e-11 426.49167073556 -1405.35625388026;-0.0006 -2.87748450607084e-11 447.63486520351 -1398.76525883973;-0.00056 -2.92059097459563e-11 468.67627136335 -1391.85619664179;-0.00052 -2.9630333259189e-11 489.611104580775 -1384.63063834758;-0.00048 -3.00480190901597e-11 510.434604455244 -1377.09022698677;-0.00044 -3.04588722607124e-11 531.142035902461 -1369.23667718385;-0.0004 -3.08627993463792e-11 551.728690231087 -1361.07177476834;-0.00036 -3.1259708497624e-11 572.189886213461 -1352.59737636863;-0.00032 -3.16495094607287e-11 592.520971150064 -1343.81540898983;-0.00028 -3.20321135983158e-11 612.717321927512 -1334.7278695756;-0.00024 -3.24074339095038e-11 632.774346069802 -1325.33682455404;-0.0002 -3.27753850496905e-11 652.68748278261 -1315.64440936778;-0.00016 -3.31358833499599e-11 672.45220399037 -1305.65282798848;-0.00012 -3.34888468361072e-11 692.064015365923 -1295.36435241555;-8e-05 -3.38341952472794e-11 711.518457352488 -1284.78132215964;-4e-05 -3.41718500542261e-11 730.811106177725 -1273.90614371054]  x5=0.00139688767047948  V1=ones(3,3)  V2=ones(3,3)  I1=ones(3,3)  I2=ones(3,3)  nHarmo=1  Measurements=None  Decoupling=off  VsMag0=0  VrMag0=0  VsAngle0=0  VrAngle0=0  IsMag0=0  IrMag0=0  IsAngle0=0  IrAngle0=0
      settings: AttributesFormatString=\n
  SAG7 : powerlib/Measurements/Three-Phase V-I Measurement  VoltageMeasurement=no  SetLabelV=on  LabelV=Vabc_SAG7  Vpu=on  VpuLL=off  CurrentMeasurement=no  SetLabelI=off  LabelI=Iabc_SAG7  Ipu=off  Pbase=100e6  Vbase=735e3  OutputType=Magnitude  PhasorSimulation=off  PSBequivalent=0
  Scope4 : Scope
  Scope5 : Scope
  Scope6 : Scope
  Subsystem : Subsystem
      mask Display: disp('Display\nWaveforms')
  Subsystem1 : Subsystem
      mask Display: disp('PSS_select')
  Subsystem2 : Subsystem
      settings: OpenFcn=LoadFlow_VSC
      mask Display: color('blue'),disp('Update Loadflow')
  VSC00 : GFo_Lib/2-Level LCL-filter  fn=fb  Sn=VSC01_Sn  Pn=VSC01_Pn  Udcn=VSC01_Udc_n  Time_Step=Time_Step  bridge_type=Average (no switches)  fpwm=4e3  Un1=VSC01_Un1  Un2=VSC01_Un2  Rt_pu=VSC01_Rt_pu  Lt_pu=VSC01_Lt_pu  Rm_pu=500  Lm_pu=500  Lf_pu=VSC01_Lf_pu  Rf_pu=VSC01_Rf_pu  Cf_pu=VSC01_Cf_pu  H_DC=40  Tr_PLL=VSC01_Tr_PLL  Val_Freq_Support=on  Val_gamma=on  R_percent=VSC01_R  Rv=VSC01_Rv  W_TVR=VSC01_W_LF  I_thresh_pu=1  DX_DR=5  Kp_Rvi_pu=0.676  RLCL_D=0.7  f_damping=200  I_max_pu=1.2  Tr_I_max=10  Advanced=off  gainpopup=With Inertia  f_Inertia_Less=3  zeta_Inertia_Less=1  Param_Inertia=PI  H_GFo=5  zeta_GFo=1  LFpopup=PV  P0=0.9  Q0=-0.3128  V0=1  Theta0=-17.0119
      settings: SourceProductName=VSC4SPS
  dE_set : Constant  Value=0
  powergui : powerlib/powergui  Priority=1  SimulationMode=Discrete  SampleTime=Time_Step  frequency=60  Iterations=50  frequencyindice=60  Pbase=5500000000  ErrMax=1e-6  UnitsV=kV  UnitsW=MW  buscounter=0  FunctionMessages=off  echomessages=off  EnableUseOfTLC=off  CurrentSourceSwitches=off  DisableSnubberDevices=off  DisableRonSwitches=off  DisableVfSwitches=off  DisplayEquations=off  AutomaticDiscreteSolvers=off  SolverType=Tustin/Backward Euler (TBE)  Interpol=off  ExternalGateDelay=off  methode=off  Ts=100  x0status=blocks  SPID=off  SwTol=0  HookPort=off  NonlinearTolerance=1e-4  nMaxIteration=100  ContinueOnMaxIteration=off  RestoreLinks=warning  ResistiveCurrentMeasurement=off  Frange=[0:2:500]  Ylog=off  Xlog=on  ShowGrid=off  save=off  variable=ZData  structure=0  ZoomFFT=off  StartTime=0.0  cycles=1  DisplayStyle=1  fundamental=60  FreqAxis=off  MaxFrequency=1000  frequencyindicesteady=1  RmsSteady=1  display=off
  wires:
  PSS/1 -> Subsystem1/1(In1)
  D_Pset/1 -> VSC00/2
  dE_set/1 -> VSC00/1
  Bus Selector1/3 -> Scope6/1  "<f>"
  Bus Selector1/2 -> Scope5/1  "<Q>"
  VSC00/1 -> Bus Selector1/1
  Bus Selector1/1 -> Scope4/1  "<P>"
  connections:
  QUE Load and Wind Generation/LConn3 -- MTL-QUE 5*219km/RConn3 -- Load Flow Bus2/LConn1 -- CHM-JCA 2*252km/RConn3 -- QUE7/LConn3
  MTL7/RConn1 -- MTL-QUE 5*219km/LConn1
  MTL7/RConn2 -- MTL-QUE 5*219km/LConn2
  MTL7/RConn3 -- MTL-QUE 5*219km/LConn3
  QUE Load and Wind Generation/LConn2 -- MTL-QUE 5*219km/RConn2 -- CHM-JCA 2*252km/RConn2 -- QUE7/LConn2
  QUE Load and Wind Generation/LConn1 -- MTL-QUE 5*219km/RConn1 -- CHM-JCA 2*252km/RConn1 -- QUE7/LConn1
  Cs SAG/LConn1 -- SAG7/RConn1 -- SAG 660Mvar/LConn1
  Cs SAG/LConn2 -- SAG7/RConn2 -- SAG 660Mvar/LConn2
  Cs SAG/LConn3 -- SAG7/RConn3 -- SAG 660Mvar/LConn3
  Load Flow Bus3/LConn1 -- CHM-SAG 117km/RConn3 -- SAG7/LConn3
  Cs CHMS/LConn1 -- CHM-SAG 117km/LConn1 -- North-West Network/RConn4
  Cs CHMS/LConn2 -- CHM-SAG 117km/LConn2 -- North-West Network/RConn5
  Cs CHMS/LConn3 -- CHM-SAG 117km/LConn3 -- North-West Network/RConn6
  Cs SAG/RConn1 -- SAG-MIC 247km/LConn1
  Cs SAG/RConn3 -- SAG-MIC 247km/LConn3
  Cs CHMS/RConn3 -- CHM-JCA 2*252km/LConn3
  Cs CHMS/RConn2 -- CHM-JCA 2*252km/LConn2
  Cs CHMS/RConn1 -- CHM-JCA 2*252km/LConn1
  Cs SAG/RConn2 -- SAG-MIC 247km/LConn2
  SAG7/LConn2 -- CHM-SAG 117km/RConn2
  SAG7/LConn1 -- CHM-SAG 117km/RConn1
  SAG-MIC 247km/RConn1 -- North_East Network/LConn1
  SAG-MIC 247km/RConn2 -- North_East Network/LConn2
  SAG-MIC 247km/RConn3 -- North_East Network/LConn3
  QUE7/RConn1 -- North_East Network/LConn4
  QUE7/RConn2 -- North_East Network/LConn5
  QUE7/RConn3 -- North_East Network/LConn6
  MTL7/LConn1 -- MTL Load/LConn1 -- Load Flow Bus/LConn1 -- VSC00/RConn1 -- North-West Network/RConn1
  MTL7/LConn2 -- MTL Load/LConn2 -- VSC00/RConn2 -- North-West Network/RConn2
  MTL7/LConn3 -- MTL Load/LConn3 -- VSC00/RConn3 -- North-West Network/RConn3

== system GFo_29bus/Cs CHMS ==
  note: B
  Ca : powerlib/Elements/Series RLC Branch  LConnTagsString=__new0  RConnTagsString=__new0  BranchType=C  Resistance=1.0  Inductance=1.0  SetiL0=off  InitialCurrent=0  Capacitance=Cs  Setx0=off  InitialVoltage=0  Measurements=None
  Cb : powerlib/Elements/Series RLC Branch  LConnTagsString=__new0  RConnTagsString=__new0  BranchType=C  Resistance=1.0  Inductance=1.0  SetiL0=off  InitialCurrent=0  Capacitance=Cs  Setx0=off  InitialVoltage=0  Measurements=None
  Cc : powerlib/Elements/Series RLC Branch  LConnTagsString=__new0  RConnTagsString=__new0  BranchType=C  Resistance=1.0  Inductance=1.0  SetiL0=off  InitialCurrent=0  Capacitance=Cs  Setx0=off  InitialVoltage=0  Measurements=None
  A : PMIOPort  Side=Left
  B : PMIOPort  Port=2  Side=Left
  C : PMIOPort  Port=3  Side=Left
  "A " : PMIOPort  Port=4  Side=Right
  "B " : PMIOPort  Port=5  Side=Right
  "C " : PMIOPort  Port=6  Side=Right
  connections:
  Cc/RConn1 -- "C "/RConn1
  C/RConn1 -- Cc/LConn1
  Cb/RConn1 -- "B "/RConn1
  B/RConn1 -- Cb/LConn1
  Ca/RConn1 -- "A "/RConn1
  A/RConn1 -- Ca/LConn1

== system GFo_29bus/Cs SAG ==
  note: B
  Ca : powerlib/Elements/Series RLC Branch  LConnTagsString=__new0  RConnTagsString=__new0  BranchType=C  Resistance=1.0  Inductance=1.0  SetiL0=off  InitialCurrent=0  Capacitance=Cs  Setx0=off  InitialVoltage=0  Measurements=None
  Cb : powerlib/Elements/Series RLC Branch  LConnTagsString=__new0  RConnTagsString=__new0  BranchType=C  Resistance=1.0  Inductance=1.0  SetiL0=off  InitialCurrent=0  Capacitance=Cs  Setx0=off  InitialVoltage=0  Measurements=None
  Cc : powerlib/Elements/Series RLC Branch  LConnTagsString=__new0  RConnTagsString=__new0  BranchType=C  Resistance=1.0  Inductance=1.0  SetiL0=off  InitialCurrent=0  Capacitance=Cs  Setx0=off  InitialVoltage=0  Measurements=None
  A : PMIOPort  Side=Left
  B : PMIOPort  Port=2  Side=Left
  C : PMIOPort  Port=3  Side=Left
  "A " : PMIOPort  Port=4  Side=Right
  "B " : PMIOPort  Port=5  Side=Right
  "C " : PMIOPort  Port=6  Side=Right
  connections:
  A/RConn1 -- Ca/LConn1
  Ca/RConn1 -- "A "/RConn1
  B/RConn1 -- Cb/LConn1
  Cb/RConn1 -- "B "/RConn1
  C/RConn1 -- Cc/LConn1
  Cc/RConn1 -- "C "/RConn1

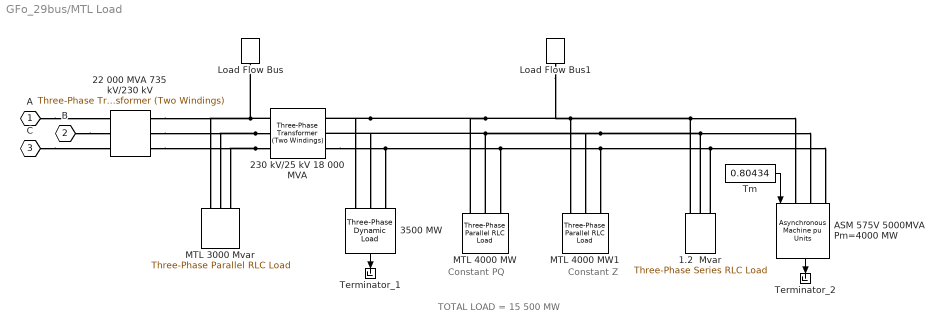
== system GFo_29bus/MTL Load ==
  note: Constant PQ
  note: Constant Z
  note: TOTAL LOAD = 15 500 MW
  1.2  Mvar : powerlib/Elements/Three-Phase Series RLC Load  LConnTagsString=A|B|C  Configuration=Y (grounded)  NominalVoltage=25e3  Vabc=[1e3 1e3 1e3]  Vabcp=[1e3 1e3 1e3]  NominalFrequency=60  UnbalancedPower=off  ActivePower=2000e6/50  InductivePower=0  CapacitivePower=2000e6  Pabc=[10e3 9e3 11e3]  QLabc=[100 90 110]  QCabc=[100 90 110]  Pabcp=[10e3 9e3 11e3]  QLabcp=[100 90 110]  QCabcp=[100 90 110]  Measurements=None  LoadType=constant Z
  22 000 MVA 735 kV/230 kV : powerlib/Elements/Three-Phase Transformer (Two Windings)  Winding1Connection=Yg  Winding2Connection=Delta (D1)  CoreType=Three single-phase transformers  SetSaturation=off  Hysteresis=off  DataFile='basic_model'  SetInitialFlux=off  Measurements=None  UNITS=pu  NominalPower=[ 22000e6 60 ]  Winding1="[ 735e3 0.002  0.12]"  Winding2=[230e3 0.002 0]  Rm=500  Lm=500  L0=0.5  Saturation="[ 0,0  ;  0.005,1.2  ;  1.0,1.4 ]"  InitialFluxes=[ 0.8 , -0.8 , 0.7 ]  BreakLoop=off  DiscreteSolver=Trapezoidal iterative  DataType=off  TransfoNumber=0
  230 kV/25 kV 18 000 MVA : powerlib/Elements/Three-Phase Transformer (Two Windings)  Winding1Connection=Yg  Winding2Connection=Delta (D1)  CoreType=Three single-phase transformers  SetSaturation=off  Hysteresis=off  DataFile='basic_model'  SetInitialFlux=off  Measurements=None  UNITS=pu  NominalPower=[18000e6 60 ]  Winding1="[ 230e3  0.08/30   0.08 ]"  Winding2="[ 25e3  0.08/30  0.08]"  Rm=500  Lm=500  L0=0.5  Saturation="[ 0,0  ;  0.005,1.2  ;  1.0,1.4 ]"  InitialFluxes=[ 0.8 , -0.8 , 0.7 ]  BreakLoop=off  DiscreteSolver=Trapezoidal iterative  DataType=off  TransfoNumber=0
  3500 MW : powerlib/Elements/Three-Phase Dynamic Load  NominalVoltage=[ 25e3 60 ]  ActiveReactivePowers=[3.5e+09 -7.63278e-08]  PositiveSequence=[0.977579 -90.0235]  ExternalControl=off  NpNq="[1.5  2.5]"  TimeConstants="[0  0  0  0]"  MinimumVoltage=0.7  Tfilter=1e-4  LoadFlowParameters=[4,0,0,0,0]
      settings: SourceProductBaseCode=PS
  ASM 575V 5000MVA Pm=4000 MW : powerlib/Machines/Asynchronous Machine pu Units  RotorType=Squirrel-cage  PresetModel=No  MechanicalLoad=Torque Tm  ShowDetailedParameters=on  ReferenceFrame=Rotor  Units=pu  MeasurementBus=off  NominalParameters="[5000e6 25e3  60]"  Stator=[0.01117 0.04832]  Rotor=[0.006 0.04832]  Cage1=[0.01909 0.0397]  Cage2=[0.01909 0.0397]  Lm=2.424  Mechanical="[1  0   2]"  PolePairs=2  InitialConditions=[0.00539423 0 0.951058 0.951058 0.951058 -118.861 -238.861 1.13934]  SimulateSaturation=off  Saturation="[0.212,0.4201,0.8125,1.0979,1.4799,2.2457,3.2586,4.5763,6.4763 ;   0.5,0.7,0.9,1,1.1,1.2 ,1.3,1.4,1.5]"  LoadFlowParameters=0  TsPowergui=0  TsBlock=-1  IterativeModel=Trapezoidal non iterative  IterativeDiscreteModel=Trapezoidal non iterative  Pmec=4000000000
      settings: SourceProductBaseCode=PS
  Load Flow Bus : powerlib/Measurements/Load Flow Bus  LConnTagsString=a  Phases=single  Connectors=on one side  ID=MTL2  Vbase=230e3  Vref=1  Vangle=0  VLF=0.9954  VLFb=1  VLFc=1  angleLF=-51.92  angleLFb=0  angleLFc=0
      settings: AttributesFormatString=%<ID>\n%<Vbase>V\n%<VLF>pu\n%<angleLF>deg.
  Load Flow Bus1 : powerlib/Measurements/Load Flow Bus  LConnTagsString=a  Phases=single  Connectors=on one side  ID=MTL_25  Vbase=25e3  Vref=1  Vangle=0  VLF=0.9776  VLFb=1  VLFc=1  angleLF=-90.02  angleLFb=0  angleLFc=0
      settings: AttributesFormatString=%<ID>\n%<Vbase>V\n%<VLF>pu\n%<angleLF>deg.
  MTL 3000 Mvar : powerlib/Elements/Three-Phase Parallel RLC Load  LConnTagsString=A|B|C  Configuration=Y (grounded)  NominalVoltage=230e3  Vabc=[1e3 1e3 1e3]  Vabcp=[1e3 1e3 1e3]  NominalFrequency=60  UnbalancedPower=off  ActivePower=0  InductivePower=0  CapacitivePower=3000e6  Pabc=[10e3 9e3 11e3]  QLabc=[100 90 110]  QCabc=[100 90 110]  Pabcp=[10e3 9e3 11e3]  QLabcp=[100 90 110]  QCabcp=[100 90 110]  Measurements=None  LoadType=constant Z
  MTL 4000 MW : powerlib/Elements/Three-Phase Parallel RLC Load  LConnTagsString=A|B|C  Configuration=Y (grounded)  NominalVoltage=(25000)*0.977579  Vabc=[1e3 1e3 1e3]  Vabcp=[1e3 1e3 1e3]  NominalFrequency=60  UnbalancedPower=off  ActivePower=4000000000  InductivePower=0  CapacitivePower=0  Pabc=[10e3 9e3 11e3]  QLabc=[100 90 110]  QCabc=[100 90 110]  Pabcp=[10e3 9e3 11e3]  QLabcp=[100 90 110]  QCabcp=[100 90 110]  Measurements=None  LoadType=constant PQ
  MTL 4000 MW1 : powerlib/Elements/Three-Phase Parallel RLC Load  LConnTagsString=A|B|C  Configuration=Y (grounded)  NominalVoltage=25e3  Vabc=[1e3 1e3 1e3]  Vabcp=[1e3 1e3 1e3]  NominalFrequency=60  UnbalancedPower=off  ActivePower=4000000000  InductivePower=0  CapacitivePower=0  Pabc=[10e3 9e3 11e3]  QLabc=[100 90 110]  QCabc=[100 90 110]  Pabcp=[10e3 9e3 11e3]  QLabcp=[100 90 110]  QCabcp=[100 90 110]  Measurements=None  LoadType=constant Z
  Terminator_1 : Terminator
  Terminator_2 : Terminator
  Tm : Constant  Value=0.80434
  A : PMIOPort  Side=Left
  B : PMIOPort  Port=2  Side=Left
  C : PMIOPort  Port=3  Side=Left
  wires:
  Tm/1 -> ASM 575V 5000MVA Pm=4000 MW/1
  3500 MW/1 -> Terminator_1/1
  ASM 575V 5000MVA Pm=4000 MW/1 -> Terminator_2/1
  connections:
  A/RConn1 -- 22 000 MVA 735 kV/230 kV/LConn1
  B/RConn1 -- 22 000 MVA 735 kV/230 kV/LConn2
  C/RConn1 -- 22 000 MVA 735 kV/230 kV/LConn3
  230 kV/25 kV 18 000 MVA/LConn1 -- Load Flow Bus/LConn1 -- 22 000 MVA 735 kV/230 kV/RConn1 -- MTL 3000 Mvar/LConn1
  230 kV/25 kV 18 000 MVA/LConn2 -- 22 000 MVA 735 kV/230 kV/RConn2 -- MTL 3000 Mvar/LConn2
  230 kV/25 kV 18 000 MVA/LConn3 -- 22 000 MVA 735 kV/230 kV/RConn3 -- MTL 3000 Mvar/LConn3
  MTL 4000 MW1/LConn1 -- Load Flow Bus1/LConn1 -- MTL 4000 MW/LConn1 -- 230 kV/25 kV 18 000 MVA/RConn1 -- 3500 MW/LConn1 -- ASM 575V 5000MVA Pm=4000 MW/LConn1 -- 1.2  Mvar/LConn1
  MTL 4000 MW1/LConn2 -- MTL 4000 MW/LConn2 -- 230 kV/25 kV 18 000 MVA/RConn2 -- 3500 MW/LConn2 -- ASM 575V 5000MVA Pm=4000 MW/LConn2 -- 1.2  Mvar/LConn2
  230 kV/25 kV 18 000 MVA/RConn3 -- ASM 575V 5000MVA Pm=4000 MW/LConn3 -- 1.2  Mvar/LConn3 -- MTL 4000 MW1/LConn3 -- MTL 4000 MW/LConn3 -- 3500 MW/LConn3

== system GFo_29bus/Model Initialization ==
